simulink model "SimulationResults"  (R2016b)
settings: Solver=FixedStepAuto  StartTime=0.0  StopTime=t  FixedStep=0.05  RelTol=1e-3
model workspace (MAT data in the model file):
  index = Simulink.Signal
  index.DataType = 'double'
  index.Dimensions = 1
  index.DimensionsMode = 'Fixed'
  index.Complexity = 'real'
  index.SampleTime = -1
  index.SamplingMode = 'auto'
  index.InitialValue = '1'
values from neighbouring files (symbols this model uses):
  AcceptRadius = 1    [Parameters.m]
  dx = 2.86    [Parameters.m]
  dy = 32.5    [Parameters.m]
  dyaw = 0.22285    [Parameters.m]
  enable_disturbance = 1    [PlannerResults.m]
  Iz = 1.10675    [Parameters.m]
  l1 = 0.05    [Parameters.m]
  l2 = 0.05    [Parameters.m]
  m = 13    [Parameters.m]
  noise_power_xbdot = 0    [PlannerResults.m]
  noise_power_yaw = 0    [PlannerResults.m]
  noise_power_yawdot = 0    [PlannerResults.m]
  refXdot = 0.5    [PlannerResults.m]
  sineAmplitude = 1    [PlannerResults.m]
  sineFrequency = 10    [PlannerResults.m]
  Ts = 0.05    [Parameters.m]
  wps = [wps ... (first row only)    [pathGeneration.m]
  xbDisturbance = 1.5    [PlannerResults.m]
  yawDisturbance = 1.5    [PlannerResults.m]
  ybDisturbance = 1.5    [PlannerResults.m]
undefined symbols (not defined in the file or in its folder): DiscIntNeverNeededParam, F_lqr, F_rob, FI_lqr, FI_rob
libraries: simulink x6
settings Model: Creator=USUARIO  LastModifiedBy=USUARIO
settings DataIOCC: Refine=100

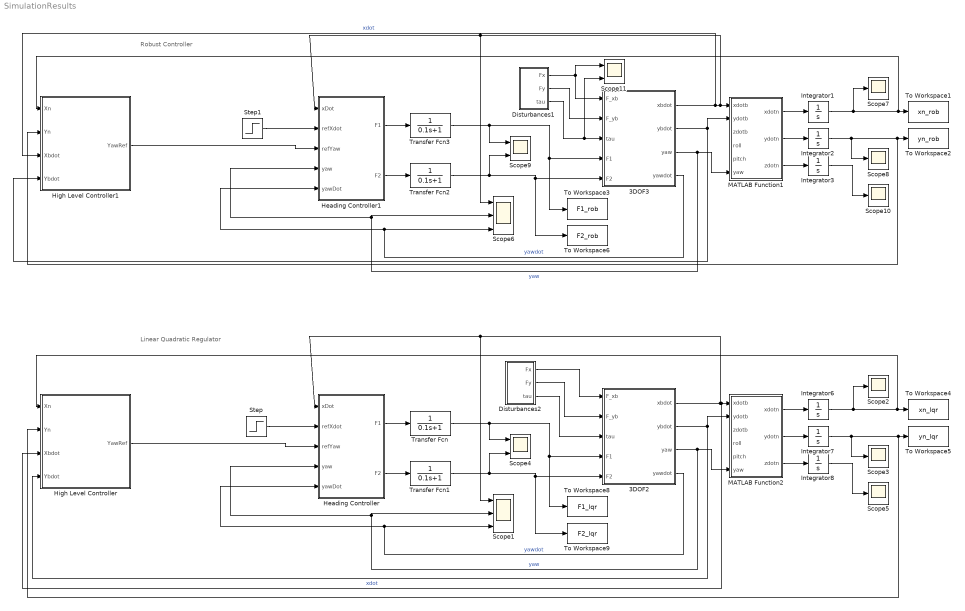
== system SimulationResults ==
  note: Linear Quadratic Regulator
  note: Robust Controller
  3DOF2 : Subsystem
  3DOF3 : Subsystem
  Disturbances1 : Subsystem
  Disturbances2 : Subsystem
  Heading Controller : Subsystem
  Heading Controller1 : Subsystem
  High Level Controller : Subsystem
  High Level Controller1 : Subsystem
  Integrator{1..3,6..8} (6 alike) : Integrator
  MATLAB Function1 : MATLAB Function  TreatAsAtomicUnit=on
  MATLAB Function2 : MATLAB Function  TreatAsAtomicUnit=on
  Scope1 : Scope  NumInputPorts=3
  Scope{2..3,5,7..8,10} (6 alike) : Scope
  Scope11 : Scope  NumInputPorts=2
  Scope4 : Scope  NumInputPorts=2
  Scope6 : Scope  NumInputPorts=3
  Scope9 : Scope  NumInputPorts=2
  Step : Step  Time=0  After=refXdot  SampleTime=0
  Step1 : Step  Time=0  After=refXdot  SampleTime=0
  To Workspace1 : ToWorkspace  VariableName=xn_rob  SaveFormat=Timeseries  SampleTime=-1
  To Workspace2 : ToWorkspace  VariableName=yn_rob  SaveFormat=Timeseries  SampleTime=-1
  To Workspace3 : ToWorkspace  VariableName=F1_rob  SaveFormat=Timeseries  SampleTime=-1
  To Workspace4 : ToWorkspace  VariableName=xn_lqr  SaveFormat=Timeseries  SampleTime=-1
  To Workspace5 : ToWorkspace  VariableName=yn_lqr  SaveFormat=Timeseries  SampleTime=-1
  To Workspace6 : ToWorkspace  VariableName=F2_rob  SaveFormat=Timeseries  SampleTime=-1
  To Workspace8 : ToWorkspace  VariableName=F1_lqr  SaveFormat=Timeseries  SampleTime=-1
  To Workspace9 : ToWorkspace  VariableName=F2_lqr  SaveFormat=Timeseries  SampleTime=-1
  Transfer Fcn{,1..3} (4 alike) : TransferFcn  Denominator=[0.1 1]
  wires:
  3DOF2/1(xbdot) -> Scope1/1, Heading Controller/1(xDot), High Level Controller/3(Xbdot), MATLAB Function2/1(xdotb)  "xdot"
  3DOF2/2(ybdot) -> High Level Controller/4("Ybdot "), MATLAB Function2/2(ydotb)
  3DOF2/3(yaw) -> MATLAB Function2/6(yaw), Scope1/2, Heading Controller/4(yaw)  "yaw"
  Integrator6/1 -> Scope2/1, High Level Controller/1(Xn), To Workspace4/1
  Integrator7/1 -> Scope3/1, High Level Controller/2(Yn), To Workspace5/1
  MATLAB Function2/3(zdotn) -> Integrator8/1
  3DOF2/4(yawdot) -> Heading Controller/5(yawDot), Scope1/3  "yawdot"
  Heading Controller/2(F2) -> Transfer Fcn1/1
  Heading Controller/1(F1) -> Transfer Fcn/1
  MATLAB Function2/1(xdotn) -> Integrator6/1
  MATLAB Function2/2(ydotn) -> Integrator7/1
  Integrator8/1 -> Scope5/1
  High Level Controller/1(YawRef) -> Heading Controller/3(refYaw)
  Step/1 -> Heading Controller/2(refXdot)
  3DOF3/3(yaw) -> Scope6/2, Heading Controller1/4(yaw), MATLAB Function1/6(yaw)  "yaw"
  MATLAB Function1/3(zdotn) -> Integrator3/1
  3DOF3/4(yawdot) -> Scope6/3, Heading Controller1/5(yawDot)  "yawdot"
  Heading Controller1/2(F2) -> Transfer Fcn2/1
  Heading Controller1/1(F1) -> Transfer Fcn3/1
  MATLAB Function1/1(xdotn) -> Integrator1/1
  MATLAB Function1/2(ydotn) -> Integrator2/1
  Integrator3/1 -> Scope10/1
  Transfer Fcn/1 -> Scope4/1, 3DOF2/4(F1), To Workspace8/1
  Transfer Fcn1/1 -> Scope4/2, 3DOF2/5(F2), To Workspace9/1
  Transfer Fcn2/1 -> 3DOF3/5(F2), To Workspace6/1, Scope9/2
  Transfer Fcn3/1 -> 3DOF3/4(F1), To Workspace3/1, Scope9/1
  Disturbances1/1(Fx) -> 3DOF3/1(F_xb), Scope11/1
  Disturbances1/3(tau) -> Scope11/2, 3DOF3/3(tau)
  Disturbances2/1(Fx) -> 3DOF2/1(F_xb)
  Disturbances2/3(tau) -> 3DOF2/3(tau)
  3DOF3/1(xbdot) -> High Level Controller1/3(Xbdot), MATLAB Function1/1(xdotb), Scope6/1, Heading Controller1/1(xDot)  "xdot"
  3DOF3/2(ybdot) -> High Level Controller1/4("Ybdot "), MATLAB Function1/2(ydotb)
  Integrator1/1 -> High Level Controller1/1(Xn), To Workspace1/1, Scope7/1
  Integrator2/1 -> High Level Controller1/2(Yn), To Workspace2/1, Scope8/1
  High Level Controller1/1(YawRef) -> Heading Controller1/3(refYaw)
  Step1/1 -> Heading Controller1/2(refXdot)
  Disturbances1/2(Fy) -> 3DOF3/2(F_yb)
  Disturbances2/2(Fy) -> 3DOF2/2(F_yb)

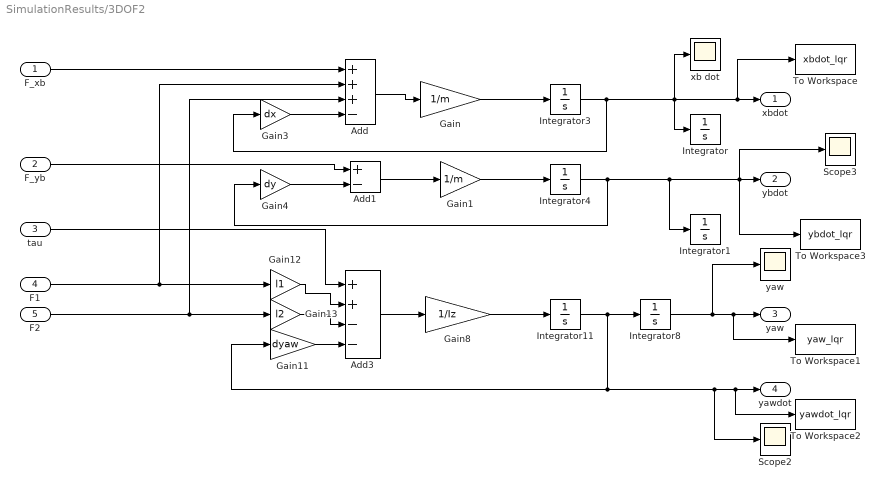
== system SimulationResults/3DOF2 ==
  F_xb : Inport
  F_yb : Inport  Port=2
  tau : Inport  Port=3
  F1 : Inport  Port=4
  F2 : Inport  Port=5
  Add : Sum  Inputs=+++-
  Add1 : Sum  Inputs=+-
  Add3 : Sum  Inputs=++--
  Gain : Gain  Gain=1/m
  Gain1 : Gain  Gain=1/m
  Gain11 : Gain  Gain=dyaw
  Gain12 : Gain  Gain=l1
  Gain13 : Gain  Gain=l2
  Gain3 : Gain  Gain=dx
  Gain4 : Gain  Gain=dy
  Gain8 : Gain  Gain=1/Iz
  Integrator{,1,3..4,8,11} (6 alike) : Integrator
  Scope2 : Scope
  Scope3 : Scope
  To Workspace : ToWorkspace  VariableName=xbdot_lqr  SaveFormat=Timeseries  SampleTime=Ts
  To Workspace1 : ToWorkspace  VariableName=yaw_lqr  SaveFormat=Timeseries  SampleTime=Ts
  To Workspace2 : ToWorkspace  VariableName=yawdot_lqr  SaveFormat=Timeseries  SampleTime=Ts
  To Workspace3 : ToWorkspace  VariableName=ybdot_lqr  SaveFormat=Timeseries  SampleTime=Ts
  xb dot : Scope
  "yaw " : Scope
  xbdot : Outport
  ybdot : Outport  Port=2
  yaw : Outport  Port=3
  yawdot : Outport  Port=4
  wires:
  Integrator11/1 -> Scope2/1, To Workspace2/1, yawdot/1, Gain11/1, Integrator8/1
  Gain8/1 -> Integrator11/1
  Gain4/1 -> Add1/2
  Gain1/1 -> Integrator4/1
  Gain3/1 -> Add/4
  Add/1 -> Gain/1
  Gain/1 -> Integrator3/1
  Gain12/1 -> Add3/2
  Add3/1 -> Gain8/1
  Gain11/1 -> Add3/4
  Gain13/1 -> Add3/3
  Integrator3/1 -> xb dot/1, Integrator/1, To Workspace/1, xbdot/1, Gain3/1
  Integrator4/1 -> Gain4/1, Integrator1/1, To Workspace3/1, ybdot/1, Scope3/1
  Integrator8/1 -> "yaw "/1, To Workspace1/1, yaw/1
  F1/1 -> Add/2, Gain12/1
  F2/1 -> Add/3, Gain13/1
  Add1/1 -> Gain1/1
  F_yb/1 -> Add1/1
  F_xb/1 -> Add/1
  tau/1 -> Add3/1

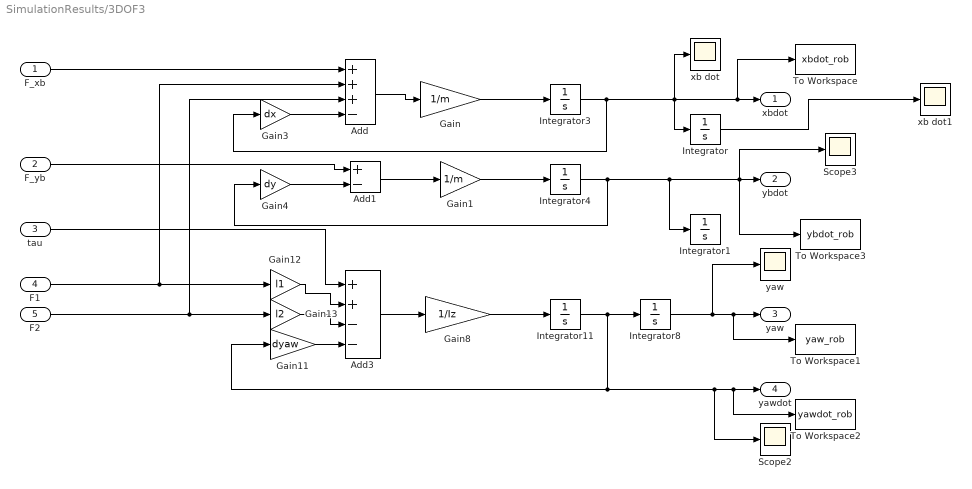
== system SimulationResults/3DOF3 ==
  F_xb : Inport
  F_yb : Inport  Port=2
  tau : Inport  Port=3
  F1 : Inport  Port=4
  F2 : Inport  Port=5
  Add : Sum  Inputs=+++-
  Add1 : Sum  Inputs=+-
  Add3 : Sum  Inputs=++--
  Gain : Gain  Gain=1/m
  Gain1 : Gain  Gain=1/m
  Gain11 : Gain  Gain=dyaw
  Gain12 : Gain  Gain=l1
  Gain13 : Gain  Gain=l2
  Gain3 : Gain  Gain=dx
  Gain4 : Gain  Gain=dy
  Gain8 : Gain  Gain=1/Iz
  Integrator{,1,3..4,8,11} (6 alike) : Integrator
  Scope2 : Scope
  Scope3 : Scope
  To Workspace : ToWorkspace  VariableName=xbdot_rob  SaveFormat=Timeseries  SampleTime=Ts
  To Workspace1 : ToWorkspace  VariableName=yaw_rob  SaveFormat=Timeseries  SampleTime=Ts
  To Workspace2 : ToWorkspace  VariableName=yawdot_rob  SaveFormat=Timeseries  SampleTime=Ts
  To Workspace3 : ToWorkspace  VariableName=ybdot_rob  SaveFormat=Timeseries  SampleTime=Ts
  xb dot : Scope
  xb dot1 : Scope
  "yaw " : Scope
  xbdot : Outport
  ybdot : Outport  Port=2
  yaw : Outport  Port=3
  yawdot : Outport  Port=4
  wires:
  tau/1 -> Add3/1
  F_xb/1 -> Add/1
  F_yb/1 -> Add1/1
  Add1/1 -> Gain1/1
  F2/1 -> Gain13/1, Add/3
  F1/1 -> Gain12/1, Add/2
  Integrator8/1 -> yaw/1, To Workspace1/1, "yaw "/1
  Integrator4/1 -> Scope3/1, ybdot/1, To Workspace3/1, Integrator1/1, Gain4/1
  Integrator3/1 -> Gain3/1, xbdot/1, To Workspace/1, Integrator/1, xb dot/1
  Gain13/1 -> Add3/3
  Gain11/1 -> Add3/4
  Add3/1 -> Gain8/1
  Gain12/1 -> Add3/2
  Gain/1 -> Integrator3/1
  Add/1 -> Gain/1
  Gain3/1 -> Add/4
  Gain1/1 -> Integrator4/1
  Gain4/1 -> Add1/2
  Gain8/1 -> Integrator11/1
  Integrator11/1 -> Integrator8/1, Gain11/1, To Workspace2/1, yawdot/1, Scope2/1
  Integrator/1 -> xb dot1/1

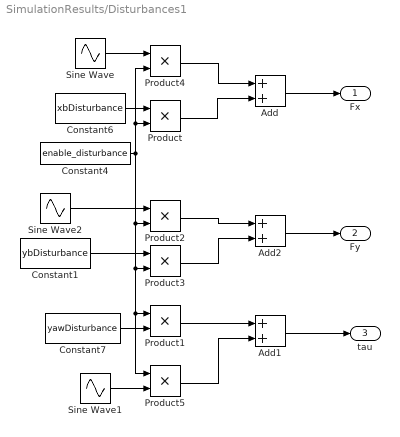
== system SimulationResults/Disturbances1 ==
  Add : Sum
  Add1 : Sum
  Add2 : Sum
  Constant1 : Constant  Value=ybDisturbance
  Constant4 : Constant  Value=enable_disturbance
  Constant6 : Constant  Value=xbDisturbance
  Constant7 : Constant  Value=yawDisturbance
  Product{,1..5} (6 alike) : Product
  Sine Wave : Sin  Amplitude=sineAmplitude  Frequency=sineFrequency  SampleTime=0
  Sine Wave1 : Sin  Amplitude=sineAmplitude  Frequency=sineFrequency  SampleTime=0
  Sine Wave2 : Sin  Amplitude=sineAmplitude  Frequency=sineFrequency  SampleTime=0
  Fx : Outport
  Fy : Outport  Port=2
  tau : Outport  Port=3
  wires:
  Product4/1 -> Add/1
  Product1/1 -> Add1/1
  Add1/1 -> tau/1
  Add/1 -> Fx/1
  Product5/1 -> Add1/2
  Sine Wave1/1 -> Product5/2
  Sine Wave/1 -> Product4/1
  Constant6/1 -> Product/1
  Product/1 -> Add/2
  Constant7/1 -> Product1/2
  Constant4/1 -> Product/2, Product4/2, Product2/2, Product3/2, Product1/1, Product5/1
  Add2/1 -> Fy/1
  Product3/1 -> Add2/2
  Product2/1 -> Add2/1
  Constant1/1 -> Product3/1
  Sine Wave2/1 -> Product2/1

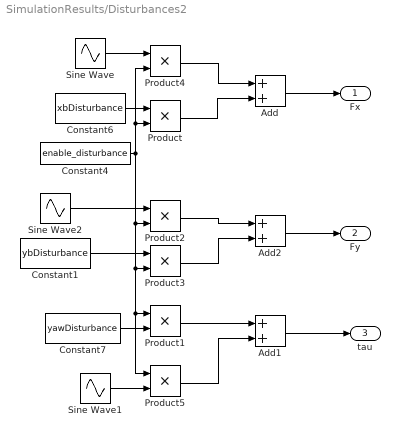
== system SimulationResults/Disturbances2 ==
  Add : Sum
  Add1 : Sum
  Add2 : Sum
  Constant1 : Constant  Value=ybDisturbance
  Constant4 : Constant  Value=enable_disturbance
  Constant6 : Constant  Value=xbDisturbance
  Constant7 : Constant  Value=yawDisturbance
  Product{,1..5} (6 alike) : Product
  Sine Wave : Sin  Amplitude=sineAmplitude  Frequency=sineFrequency  SampleTime=0
  Sine Wave1 : Sin  Amplitude=sineAmplitude  Frequency=sineFrequency  SampleTime=0
  Sine Wave2 : Sin  Amplitude=sineAmplitude  Frequency=sineFrequency  SampleTime=0
  Fx : Outport
  Fy : Outport  Port=2
  tau : Outport  Port=3
  wires:
  Product4/1 -> Add/1
  Product1/1 -> Add1/1
  Add1/1 -> tau/1
  Add/1 -> Fx/1
  Product5/1 -> Add1/2
  Sine Wave1/1 -> Product5/2
  Sine Wave/1 -> Product4/1
  Constant6/1 -> Product/1
  Product/1 -> Add/2
  Constant7/1 -> Product1/2
  Constant4/1 -> Product/2, Product4/2, Product2/2, Product3/2, Product1/1, Product5/1
  Add2/1 -> Fy/1
  Product3/1 -> Add2/2
  Product2/1 -> Add2/1
  Constant1/1 -> Product3/1
  Sine Wave2/1 -> Product2/1

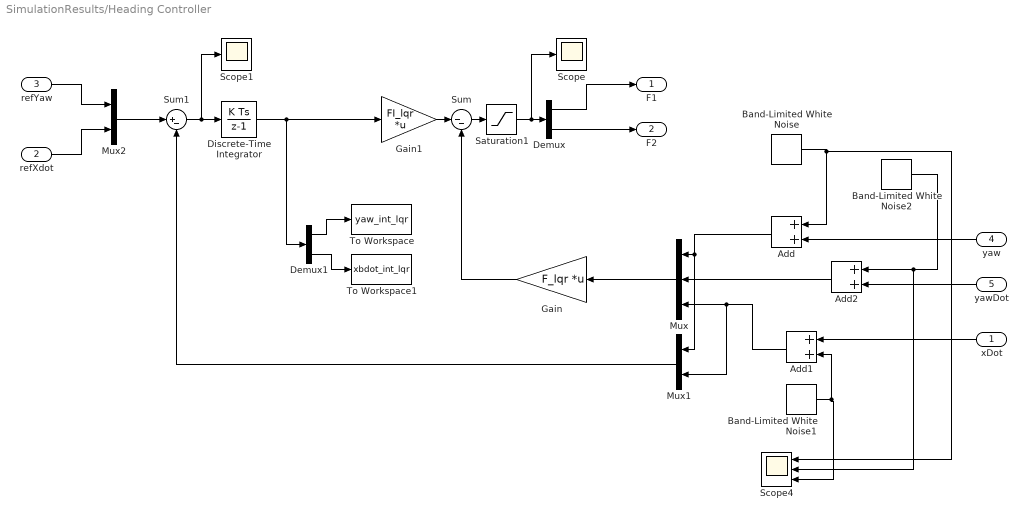
== system SimulationResults/Heading Controller ==
  xDot : Inport
  refXdot : Inport  Port=2  PortDimensions=1
  refYaw : Inport  Port=3  PortDimensions=1
  yaw : Inport  Port=4
  yawDot : Inport  Port=5
  Add : Sum
  Add1 : Sum
  Add2 : Sum
  Band-Limited White Noise : simulink/Sources/Band-Limited White Noise  Cov=[noise_power_yaw]  Ts=0.05  seed=[23341]
  Band-Limited White Noise1 : simulink/Sources/Band-Limited White Noise  Cov=[noise_power_xbdot]  Ts=0.05  seed=[23041]
  Band-Limited White Noise2 : simulink/Sources/Band-Limited White Noise  Cov=[noise_power_yawdot]  Ts=0.05  seed=[23026]
  Demux : Demux  Outputs=2
  Demux1 : Demux  Outputs=2
  Discrete-Time Integrator : DiscreteIntegrator  InitialConditionSetting=State (most efficient)  SampleTime=-1  ICPrevOutput=DiscIntNeverNeededParam  ICPrevScaledInput=DiscIntNeverNeededParam
  Gain : Gain  Gain=F_lqr  Multiplication=Matrix(K*u)
  Gain1 : Gain  Gain=FI_lqr  Multiplication=Matrix(K*u)
  Mux : Mux  Inputs=3
  Mux1 : Mux  Inputs=2
  Mux2 : Mux  Inputs=2
  Saturation1 : Saturate  UpperLimit=50  LowerLimit=-25
  Scope : Scope
  Scope1 : Scope
  Scope4 : Scope  NumInputPorts=3
  Sum : Sum  Inputs=|--
  Sum1 : Sum  Inputs=|+-
  To Workspace : ToWorkspace  VariableName=yaw_int_lqr  SaveFormat=Timeseries  SampleTime=-1
  To Workspace1 : ToWorkspace  VariableName=xbdot_int_lqr  SaveFormat=Timeseries  SampleTime=-1
  F1 : Outport
  F2 : Outport  Port=2
  wires:
  Saturation1/1 -> Scope/1, Demux/1
  Sum1/1 -> Scope1/1, Discrete-Time Integrator/1
  Demux/1 -> F1/1
  Demux/2 -> F2/1
  Sum/1 -> Saturation1/1
  Gain/1 -> Sum/2
  Mux/1 -> Gain/1
  refYaw/1 -> Mux2/1
  Mux2/1 -> Sum1/1
  Mux1/1 -> Sum1/2
  refXdot/1 -> Mux2/2
  Gain1/1 -> Sum/1
  Discrete-Time Integrator/1 -> Demux1/1, Gain1/1
  Demux1/1 -> To Workspace/1
  Demux1/2 -> To Workspace1/1
  Add1/1 -> Mux/3, Mux1/2
  Band-Limited White Noise1/1 -> Scope4/3, Add1/2
  xDot/1 -> Add1/1
  Band-Limited White Noise/1 -> Scope4/1, Add/1
  yaw/1 -> Add/2
  yawDot/1 -> Add2/2
  Add/1 -> Mux/1, Mux1/1
  Add2/1 -> Mux/2
  Band-Limited White Noise2/1 -> Scope4/2, Add2/1

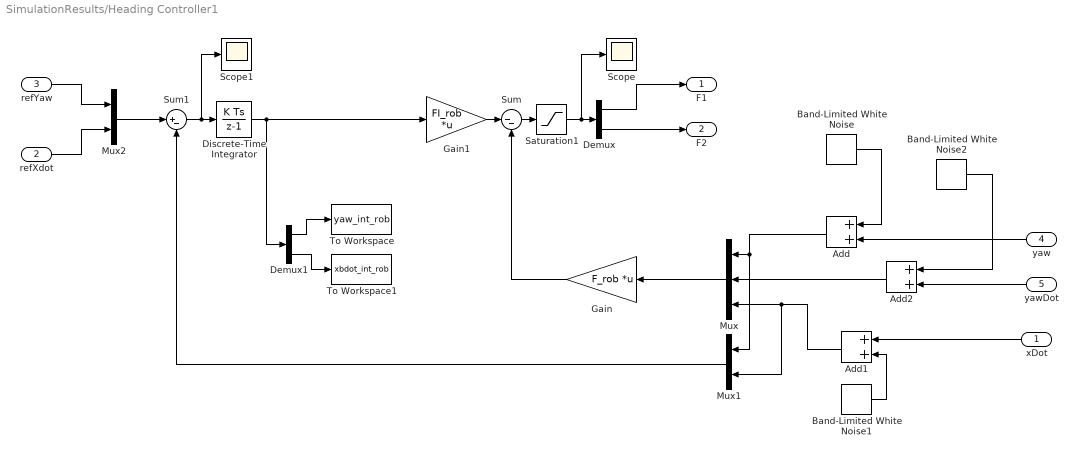
== system SimulationResults/Heading Controller1 ==
  xDot : Inport
  refXdot : Inport  Port=2  PortDimensions=1
  refYaw : Inport  Port=3  PortDimensions=1
  yaw : Inport  Port=4
  yawDot : Inport  Port=5
  Add : Sum
  Add1 : Sum
  Add2 : Sum
  Band-Limited White Noise : simulink/Sources/Band-Limited White Noise  Cov=[noise_power_yaw]  Ts=0.05  seed=[23341]
  Band-Limited White Noise1 : simulink/Sources/Band-Limited White Noise  Cov=[noise_power_xbdot]  Ts=0.05  seed=[23041]
  Band-Limited White Noise2 : simulink/Sources/Band-Limited White Noise  Cov=[noise_power_yawdot]  Ts=0.05  seed=[23026]
  Demux : Demux  Outputs=2
  Demux1 : Demux  Outputs=2
  Discrete-Time Integrator : DiscreteIntegrator  InitialConditionSetting=State (most efficient)  SampleTime=-1  ICPrevOutput=DiscIntNeverNeededParam  ICPrevScaledInput=DiscIntNeverNeededParam
  Gain : Gain  Gain=F_rob  Multiplication=Matrix(K*u)
  Gain1 : Gain  Gain=FI_rob  Multiplication=Matrix(K*u)
  Mux : Mux  Inputs=3
  Mux1 : Mux  Inputs=2
  Mux2 : Mux  Inputs=2
  Saturation1 : Saturate  UpperLimit=50  LowerLimit=-25
  Scope : Scope
  Scope1 : Scope
  Sum : Sum  Inputs=|--
  Sum1 : Sum  Inputs=|+-
  To Workspace : ToWorkspace  VariableName=yaw_int_rob  SaveFormat=Timeseries  SampleTime=-1
  To Workspace1 : ToWorkspace  VariableName=xbdot_int_rob  SaveFormat=Timeseries  SampleTime=-1
  F1 : Outport
  F2 : Outport  Port=2
  wires:
  Gain1/1 -> Sum/1
  Add1/1 -> Mux1/2, Mux/3
  Band-Limited White Noise1/1 -> Add1/2
  xDot/1 -> Add1/1
  Band-Limited White Noise/1 -> Add/1
  yaw/1 -> Add/2
  refXdot/1 -> Mux2/2
  Mux1/1 -> Sum1/2
  Mux2/1 -> Sum1/1
  refYaw/1 -> Mux2/1
  Mux/1 -> Gain/1
  Gain/1 -> Sum/2
  Sum/1 -> Saturation1/1
  yawDot/1 -> Add2/2
  Discrete-Time Integrator/1 -> Demux1/1, Gain1/1
  Demux/2 -> F2/1
  Demux/1 -> F1/1
  Sum1/1 -> Scope1/1, Discrete-Time Integrator/1
  Add/1 -> Mux/1, Mux1/1
  Saturation1/1 -> Demux/1, Scope/1
  Demux1/1 -> To Workspace/1
  Demux1/2 -> To Workspace1/1
  Add2/1 -> Mux/2
  Band-Limited White Noise2/1 -> Add2/1

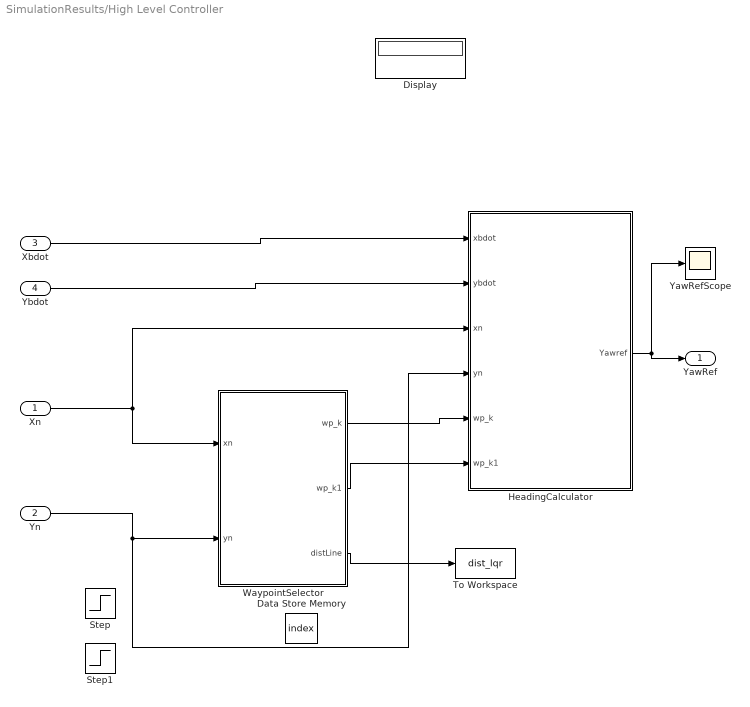
== system SimulationResults/High Level Controller ==
  Xn : Inport  OutDataTypeStr=double  PortDimensions=1
  Yn : Inport  Port=2  OutDataTypeStr=double  PortDimensions=1
  Xbdot : Inport  Port=3  OutDataTypeStr=double  PortDimensions=1
  "Ybdot " : Inport  Port=4  OutDataTypeStr=double  PortDimensions=1
  Data Store Memory : DataStoreMemory  DataStoreName=index  ReadBeforeWriteMsg=warning  WriteAfterWriteMsg=warning  WriteAfterReadMsg=warning  InitialValue=1  ShowAdditionalParam=off  OutDataTypeStr=double  Dimensions=1
  Display : Display
  HeadingCalculator : MATLAB Function  TreatAsAtomicUnit=on
  Step : Step  Time=200  Before=1  After=-101  SampleTime=0
  Step1 : Step  Time=200  Before=1  After=25  SampleTime=0
  To Workspace : ToWorkspace  VariableName=dist_lqr  SaveFormat=Timeseries  SampleTime=-1
  WaypointSelector : MATLAB Function  TreatAsAtomicUnit=on
  YawRefScope : Scope
  YawRef : Outport
  wires:
  Xn/1 -> WaypointSelector/1(xn), HeadingCalculator/3(xn)
  Yn/1 -> HeadingCalculator/4(yn), WaypointSelector/2(yn)
  HeadingCalculator/1(Yawref) -> YawRef/1, YawRefScope/1
  WaypointSelector/1(wp_k) -> HeadingCalculator/5(wp_k)
  WaypointSelector/2(wp_k1) -> HeadingCalculator/6(wp_k1)
  Xbdot/1 -> HeadingCalculator/1(xbdot)
  "Ybdot "/1 -> HeadingCalculator/2(ybdot)
  WaypointSelector/3(distLine) -> To Workspace/1

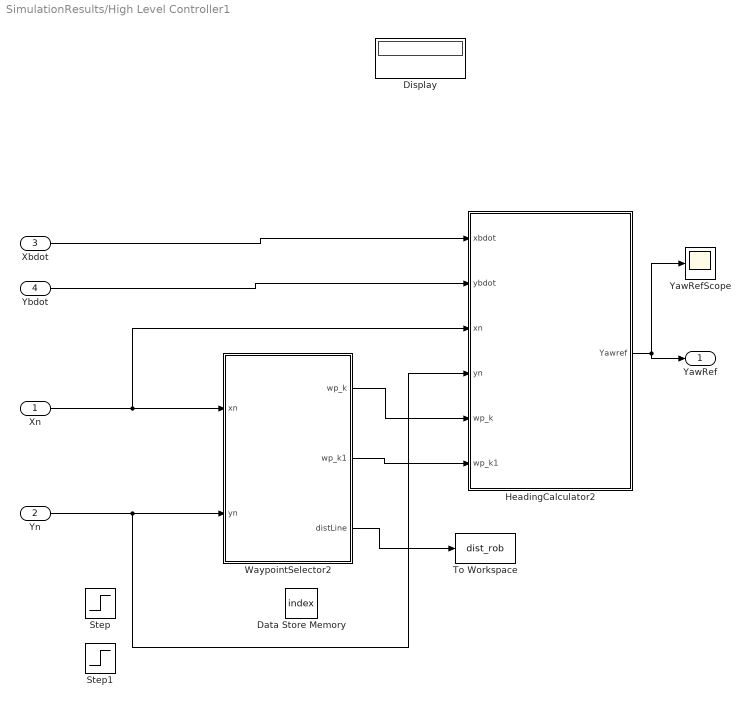
== system SimulationResults/High Level Controller1 ==
  Xn : Inport  OutDataTypeStr=double  PortDimensions=1
  Yn : Inport  Port=2  OutDataTypeStr=double  PortDimensions=1
  Xbdot : Inport  Port=3  OutDataTypeStr=double  PortDimensions=1
  "Ybdot " : Inport  Port=4  OutDataTypeStr=double  PortDimensions=1
  Data Store Memory : DataStoreMemory  DataStoreName=index  ReadBeforeWriteMsg=warning  WriteAfterWriteMsg=warning  WriteAfterReadMsg=warning  InitialValue=1  ShowAdditionalParam=off  OutDataTypeStr=double  Dimensions=1
  Display : Display
  HeadingCalculator2 : MATLAB Function  TreatAsAtomicUnit=on
  Step : Step  Time=200  Before=1  After=-101  SampleTime=0
  Step1 : Step  Time=200  Before=1  After=25  SampleTime=0
  To Workspace : ToWorkspace  VariableName=dist_rob  SaveFormat=Timeseries  SampleTime=-1
  WaypointSelector2 : MATLAB Function  TreatAsAtomicUnit=on
  YawRefScope : Scope
  YawRef : Outport
  wires:
  Xn/1 -> WaypointSelector2/1(xn), HeadingCalculator2/3(xn)
  Yn/1 -> WaypointSelector2/2(yn), HeadingCalculator2/4(yn)
  HeadingCalculator2/1(Yawref) -> YawRef/1, YawRefScope/1
  WaypointSelector2/1(wp_k) -> HeadingCalculator2/5(wp_k)
  WaypointSelector2/2(wp_k1) -> HeadingCalculator2/6(wp_k1)
  Xbdot/1 -> HeadingCalculator2/1(xbdot)
  "Ybdot "/1 -> HeadingCalculator2/2(ybdot)
  WaypointSelector2/3(distLine) -> To Workspace/1

== matlab function SimulationResults/MATLAB Function1 ==
  data: xdotb input; xdotn output; ydotb input; zdotb input; roll input; pitch input; yaw input; ydotn output; zdotn output
function [xdotn,ydotn,zdotn] = fcn(xdotb,ydotb,zdotb,roll,pitch,yaw)
R=[cos(pitch)*cos(yaw) sin(roll)*sin(pitch)*cos(yaw)-cos(roll)*sin(yaw) ...
                          cos(roll)*sin(pitch)*cos(yaw)+sin(roll)*sin(yaw);
   cos(pitch)*sin(yaw) sin(roll)*sin(pitch)*sin(yaw)+cos(roll)*cos(yaw) ...
                          cos(roll)*sin(pitch)*sin(yaw)-sin(roll)*cos(yaw);
   -sin(pitch) sin(roll)*cos(pitch) cos(roll)*cos(pitch)];

n=R*[xdotb;ydotb;zdotb];

xdotn=n(1);
ydotn=n(2);
zdotn=n(3);
end

== matlab function SimulationResults/High Level Controller1/HeadingCalculator2 ==
  data: xbdot input; ybdot input; xn input; Yawref output; yn input; wp_k input; wp_k1 input; r parameter
function Yawref  = HeadingCalculator(xbdot,ybdot,xn,yn,wp_k,wp_k1,r)

vessel_pos=[xn,yn];
LOSpoint=FindLOSpoint(wp_k,wp_k1,vessel_pos,r);
%a=abc(wp_k ,wp_k1);
%slope=(LOS(2)-yn)/(LOS(1)-xn);

b=atan2(ybdot,xbdot);
Yawref=atan2(LOSpoint(2)-yn,LOSpoint(1)-xn)-b;

== matlab function SimulationResults/MATLAB Function2 ==
  data: xdotb input; xdotn output; ydotb input; zdotb input; roll input; pitch input; yaw input; ydotn output; zdotn output
function [xdotn,ydotn,zdotn] = fcn(xdotb,ydotb,zdotb,roll,pitch,yaw)
R=[cos(pitch)*cos(yaw) sin(roll)*sin(pitch)*cos(yaw)-cos(roll)*sin(yaw) ...
                          cos(roll)*sin(pitch)*cos(yaw)+sin(roll)*sin(yaw);
   cos(pitch)*sin(yaw) sin(roll)*sin(pitch)*sin(yaw)+cos(roll)*cos(yaw) ...
                          cos(roll)*sin(pitch)*sin(yaw)-sin(roll)*cos(yaw);
   -sin(pitch) sin(roll)*cos(pitch) cos(roll)*cos(pitch)];

n=R*[xdotb;ydotb;zdotb];

xdotn=n(1);
ydotn=n(2);
zdotn=n(3);
end

== matlab function SimulationResults/High Level Controller/WaypointSelector ==
  data: xn input; wp_k output; yn input; wp_k1 output; AcceptRadius parameter; wps parameter; index data_store_memory; distLine output
function [wp_k,wp_k1,distLine] = WaypointSelector(xn,yn,AcceptRadius, wps)

global index;

wp_k=wps(index,:);
wp_k1=wps(index+1,:);

[dist,distLine]=FindDistWP(wp_k,wp_k1,[xn,yn]);
if (dist<AcceptRadius) && (size(wps,1)>(index+1))
    index=index+1;
    wp_k=wps(index,:);
    wp_k1=wps(index+1,:);
elseif (size(wps,1)==(index+1))
    xdotref=0; 
end
end

== matlab function SimulationResults/High Level Controller/HeadingCalculator ==
  data: xbdot input; ybdot input; xn input; Yawref output; yn input; wp_k input; wp_k1 input; r parameter
function Yawref  = HeadingCalculator(xbdot,ybdot,xn,yn,wp_k,wp_k1,r)

vessel_pos=[xn,yn];
LOSpoint=FindLOSpoint(wp_k,wp_k1,vessel_pos,r);
%a=abc(wp_k ,wp_k1);
%slope=(LOS(2)-yn)/(LOS(1)-xn);

b=atan2(ybdot,xbdot);
Yawref=atan2(LOSpoint(2)-yn,LOSpoint(1)-xn)-b;

== matlab function SimulationResults/High Level Controller1/WaypointSelector2 ==
  data: xn input; wp_k output; yn input; wp_k1 output; AcceptRadius parameter; wps parameter; index data_store_memory; distLine output
function [wp_k,wp_k1,distLine] = WaypointSelector(xn,yn,AcceptRadius, wps)

global index;

wp_k=wps(index,:);
wp_k1=wps(index+1,:);

[dist,distLine]=FindDistWP(wp_k,wp_k1,[xn,yn]);
if (dist<AcceptRadius) && (size(wps,1)>(index+1))
    index=index+1;
    wp_k=wps(index,:);
    wp_k1=wps(index+1,:);
elseif (size(wps,1)==(index+1))
    xdotref=0; 
end
end
